simulink model "TonosSumadosRuido"  (Simulink 7.1)
settings: Solver=ode45  StartTime=0.0  StopTime=0.02  RelTol=1e-3
libraries: dsparch4 x1
settings Model: Creator=Usuario  LastModifiedBy=Usuario

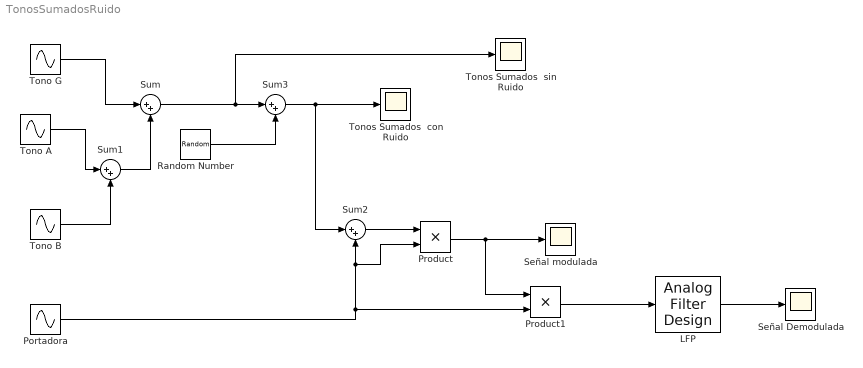
== system TonosSumadosRuido ==
  LFP : dsparch4/Analog Filter Design  method=Butterworth  filttype=Lowpass  N=10  Wlo=((392+440+494))*4  Whi=80  Rp=2  Rs=40
  Portadora : Sin  Frequency=2*pi*((392+440+494)/3)*4  SampleTime=1/44100
  Product : Product  OutDataType=sfix(16)  OutScaling=2^0  SampleTime=1/44100  RndMeth=Zero
  Product1 : Product  OutDataType=sfix(16)  OutScaling=2^0  SampleTime=1/44100  RndMeth=Zero
  Random Number : RandomNumber  SampleTime=1/44100
  Señal Demodulada : Scope
      settings: SaveName=ScopeData2
  Señal modulada : Scope
  Sum{,1..3} (4 alike) : Sum  Inputs=|++  OutDataType=sfix(16)  OutScaling=2^0  SampleTime=1/44100
  Tono A : Sin  Frequency=2*pi*440  SampleTime=1/44100
  Tono B : Sin  Frequency=2*pi*494  SampleTime=1/44100
  Tono G : Sin  Frequency=2*pi*392  SampleTime=1/44100
  Tonos Sumados  con Ruido : Scope
  Tonos Sumados  sin Ruido : Scope
      settings: SaveName=ScopeData3
  wires:
  Tono G/1 -> Sum/1
  Tono A/1 -> Sum1/1
  Tono B/1 -> Sum1/2
  Sum1/1 -> Sum/2
  Portadora/1 -> Product/2, Sum2/2, Product1/2
  Sum2/1 -> Product/1
  Product/1 -> Señal modulada/1, Product1/1
  Product1/1 -> LFP/1
  LFP/1 -> Señal Demodulada/1
  Sum/1 -> Sum3/1, Tonos Sumados  sin Ruido/1
  Random Number/1 -> Sum3/2
  Sum3/1 -> Tonos Sumados  con Ruido/1, Sum2/1
